simulink library "USVModelLib"  (R2022a)
settings: Solver=VariableStepAuto  StartTime=0.0  StopTime=10.0  RelTol=1e-3
values from neighbouring files (symbols this model uses):
  ModelParam_envAltitude = -600    [USV_init.m]
  ModelParam_noiseGPSSampTime = 0.2    [USV_init.m]
  ModelParam_noisePowerIMU = 0.0003394    [USV_init.m]
  ModelParam_timeSampBaro = 0.02    [USV_init.m]
  MotorFault1 = MotorFaultTemp    [USV_init.m]
undefined symbols (not defined in the file or in its folder): BatteryFault, Earth, ESCFault, F, FaultParamAPI, Light, LoadFault, MIL, ModelParam_noiseLowPassFilterCoeAccel, ModelParam_noiseLowPassFilterCoeGyro, Moderate, PropFault, SensorFault, WGS84, WindFault
libraries: aerolibwind2 x6, simulink x3, aerolibtransform2 x1, aerolibasang x1, aerolibatmos2 x1, aerolibnav x1, aerolibgravity2 x1
(part 2 of 2)

== matlab function USVModelLib/GPSFault/AccNoiseSwitch1/Acc NoiseFun ==
  data: u input; yNoise output; isGPSFault input; GPSFaultParams input; y3DFix output; ySats output
function [yNoise,y3DFix,ySats] = fcn(u,isGPSFault,GPSFaultParams)

yNoise = 0.3*u;
y3DFix = 3;
ySats = 10;

if isGPSFault
    yNoise = (GPSFaultParams(1))*u;
    y3DFix = GPSFaultParams(2);
    ySats = GPSFaultParams(3);
end

== matlab function USVModelLib/BatteryFault/FaultParamsExtract ==
  settings: updateMethod=DISCRETE
  data: FaultID input; inInts input; hasFault_isUseCustomHovTime output; inFloats input; FaultParam output
function [hasFault_isUseCustomHovTime, FaultParam] = fcn(FaultID,inInts,inFloats)
persistent hFault;
persistent fParam;

if isempty(hFault)
    hFault=false;
end
if isempty(fParam)
    fParam=zeros(20,1);
end

hFaultTmp=false;
fParamTmp=zeros(20,1);
j=1;
for i=1:8
    if inInts(i) == FaultID
        hFaultTmp=true;
        fParamTmp(2*j-1)=inFloats(2*i-1);
        fParamTmp(2*j)=inFloats(2*i);
        j=j+1;
    end
end
if hFaultTmp
    hFault=hFaultTmp;
    fParamTmp(17:20) = inFloats(17:20);
    fParam=fParamTmp;
end

hasFault_isUseCustomHovTime=hFault;
FaultParam=fParam;

== matlab function USVModelLib/SensorFault/FaultParamsExtract ==
  settings: updateMethod=DISCRETE
  data: FaultID input; inInts input; hasFault_acc output; inFloats input; FaultParam output
function [hasFault_acc, FaultParam] = fcn(FaultID,inInts,inFloats)
persistent hFault;
persistent fParam;

if isempty(hFault)
    hFault=false;
end
if isempty(fParam)
    fParam=zeros(20,1);
end

hFaultTmp=false;
fParamTmp=zeros(20,1);
j=1;
for i=1:8
    if inInts(i) == FaultID
        hFaultTmp=true;
        fParamTmp(2*j-1)=inFloats(2*i-1);
        fParamTmp(2*j)=inFloats(2*i);
        j=j+1;
    end
end
if hFaultTmp
    hFault=hFaultTmp;
    fParamTmp(17:20) = inFloats(17:20);
    fParam=fParamTmp;
end

hasFault_acc=hFault;
FaultParam=fParam;

== matlab function USVModelLib/SensorFault/FaultParamsExtract1 ==
  settings: updateMethod=DISCRETE
  data: FaultID input; inInts input; hasFault_gyro output; inFloats input; FaultParam output
function [hasFault_gyro, FaultParam] = fcn(FaultID,inInts,inFloats)
persistent hFault;
persistent fParam;

if isempty(hFault)
    hFault=false;
end
if isempty(fParam)
    fParam=zeros(20,1);
end

hFaultTmp=false;
fParamTmp=zeros(20,1);
j=1;
for i=1:8
    if inInts(i) == FaultID
        hFaultTmp=true;
        fParamTmp(2*j-1)=inFloats(2*i-1);
        fParamTmp(2*j)=inFloats(2*i);
        j=j+1;
    end
end
if hFaultTmp
    hFault=hFaultTmp;
    fParamTmp(17:20) = inFloats(17:20);
    fParam=fParamTmp;
end

hasFault_gyro=hFault;
FaultParam=fParam;

== matlab function USVModelLib/WindFault/MATLAB Function ==
  settings: updateMethod=DISCRETE
  data: t input; isGustWind input; gWind output; GustWindParams input; turb input
function gWind = GustWindModel(t,isGustWind,GustWindParams,turb)

if(GustWindParams(2)<1)
    GustWindParams(2)=1;
end
timeVel=60/GustWindParams(2);

vmax=GustWindParams(1);

persistent t0;
if isempty(t0)
    t0=0;
end

persistent isInGust;
if isempty(isInGust)
    isInGust=0;
end

persistent t1;
if isempty(t1)
    t1=2;
end

persistent a;
if isempty(a)
    a=0.5;
end

persistent ang;
if isempty(ang)
    ang=pi/2;
end

persistent wlast;
if isempty(wlast)
    wlast=vmax*0.5;
end

persistent wNow;
if isempty(wNow)
    wNow=1.4*0.8*vmax;
end


if isGustWind&&isInGust<0.5
    t0=t;
    t1=timeVel*(3/4+1/2*rand(1));
    a=1/4+1/2*rand(1);
    ang=pi*2*rand(1);
    wlast=wNow;
    wNow=1.2*(rand(1)*0.5+0.5)*vmax;
    
    isInGust=1;
end

if ~isGustWind
    isInGust=0;
end

gWind=[0;0;0];

if(t<t0+t1*a)
    gWindMag=(wNow-wlast)/2*(1-cos((t-t0)/(t1*a)*pi))+wlast;
else
    gWindMag=wNow;
end

if abs(t-(t0+t1))<0.05
    rng(t*1000);
    t0=t;
    t1=timeVel*(3/4+1/2*rand(1));
    a=1/4+1/2*rand(1);
    ang=ang+0.1*pi*rand(1);
    wlast=wNow;
    wNow=1.2*(rand(1)*0.5+0.5)*vmax;
end

gWind(1)=gWindMag*cos(ang)*0.8+turb(1)*0.4;
gWind(2)=gWindMag*sin(ang)*0.8+turb(2)*0.4;
gWind(3)=turb(3)*0.4;

== matlab function USVModelLib/WindFault/MATLAB Function1 ==
  data: wind output size=3; isConstWind input; isGustWind input; isTurbWind input; isSheerWind input; ConstWind input; GustWind input; TurbWind input; SheerWind input
function wind = WindFun(isConstWind,isGustWind,isTurbWind,isSheerWind,ConstWind,GustWind,TurbWind,SheerWind)
wind=[0;0;0];
if isConstWind
    wind=[ConstWind(1);ConstWind(2);ConstWind(3)];
elseif isGustWind
    wind=GustWind;
elseif isTurbWind
    wind=TurbWind;
elseif isSheerWind
    wind=SheerWind;
end

== matlab function USVModelLib/Motor Fault/FaultParamsExtract ==
  settings: updateMethod=DISCRETE
  data: FaultID input; inInts input; hasFault output; inFloats input; FaultParam output
function [hasFault, FaultParam] = fcn(FaultID,inInts,inFloats)
persistent hFault;
persistent fParam;

if isempty(hFault)
    hFault=false;
end
if isempty(fParam)
    fParam=zeros(20,1);
end

hFaultTmp=false;
fParamTmp=zeros(20,1);
j=1;
for i=1:8
    if inInts(i) == FaultID
        hFaultTmp=true;
        fParamTmp(2*j-1)=inFloats(2*i-1);
        fParamTmp(2*j)=inFloats(2*i);
        j=j+1;
    end
end
if hFaultTmp
    hFault=hFaultTmp;
    fParamTmp(17:20) = inFloats(17:20);
    fParam=fParamTmp;
end

hasFault=hFault;
FaultParam=fParam;
